simulink model "rigid_launcher_OL"  (R2020b)
settings: Solver=ode23s  StartTime=0.0  StopTime=100  FixedStep=0.05  RelTol=1e-3  EnableMultiTasking=on
undefined symbols (not defined in the file or in its folder): Ar, Br, Cr, Dr
settings Model: ExtModeAutoUpdateStatusClock=off  Creator=chiappa  LastModifiedBy=X000274
settings DataIOCC: LimitDataPoints=on  SaveFormat=Array  SignalLoggingSaveFormat=ModelDataLogs  ReturnWorkspaceOutputs=off  SignalLoggingName=sigsOut
settings OptimizationCC: BlockReduction=off  BooleanDataType=off
settings DebuggingCC: SaveWithParameterizedLinksMsg=none  UnderspecifiedInitializationDetection=Classic  MergeDetectMultiDrivingBlocksExec=none  SignalResolutionControl=TryResolveAllWithWarning  MultiTaskDSMMsg=warning  MultiTaskCondExecSysMsg=none
settings HardwareCC: ProdBitPerPointer=32  ProdBitPerSizeT=32  ProdBitPerPtrDiffT=32  ProdLargestAtomicFloat=None  ProdIntDivRoundTo=Undefined  ProdEndianess=Unspecified  ProdWordSize=32  ProdHWDeviceType=32-bit Generic  TargetUnknown=on
settings ModelReferenceCC: PropagateSignalLabelsOutOfModel=off
settings GRTTargetCC: CombineOutputUpdateFcns=off  GRTInterface=on
settings ConfigComp: CovMetricSettings=dw  CovSaveCumulativeToWorkspaceVar=on  CovSaveSingleToWorkspaceVar=on

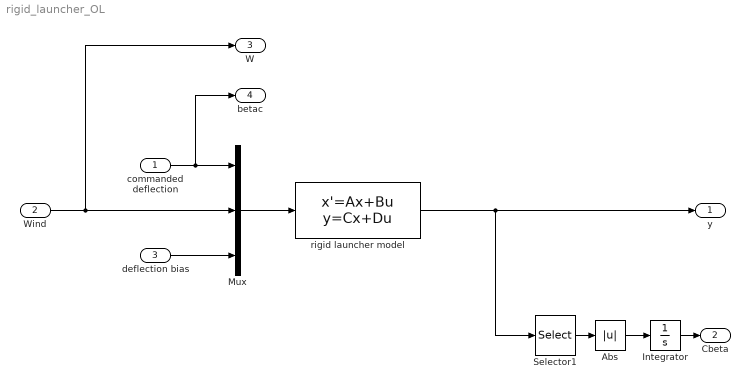
== system rigid_launcher_OL ==
  commanded deflection : Inport
  Wind : Inport  Port=2
  deflection bias : Inport  Port=3
  Abs : Abs
  Integrator : Integrator
  Mux : Mux  Inputs=3
  Selector1 : Selector  InputPortWidth=6  IndexOptions=Index vector (dialog)  Indices=[4]  OutputSizes=1
  rigid launcher model : StateSpace  A=Ar  B=Br  C=Cr  D=Dr  InitialCondition=0
  y : Outport
  Cbeta : Outport  Port=2
  W : Outport  Port=3
  betac : Outport  Port=4
  wires:
  Mux/1 -> rigid launcher model/1
  rigid launcher model/1 -> y/1, Selector1/1
  Selector1/1 -> Abs/1
  Abs/1 -> Integrator/1
  Integrator/1 -> Cbeta/1
  Wind/1 -> Mux/2, W/1
  commanded deflection/1 -> Mux/1, betac/1
  deflection bias/1 -> Mux/3
